simulink model "Discrete_time_PID"  (R2024b)
settings: Solver=ode45  StartTime=0.0  StopTime=10  RelTol=1e-3
values from neighbouring files (symbols this model uses):
  B_C = (gbox.N * mot.Ke)/drv.dcgain    [Init.m]
  Beq = 1.223604206496999e-06    (= 1.2236042065e-06)    [code_ali.m]
  den = [(TL+Ts) -TL]    [Init.m]
  F_C = mot.Req/(drv.dcgain * mot.Kt * gbox.N)    [Init.m]
  I_C = (gbox.N * mot.Req * Jeq_hat)/(drv.dcgain * mot.Kt)    [Init.m]
  Kw = 1/Tw*0.05    (= 1.66666666667)    [Init.m]
  num = [1 -1]    [Init.m]
  Ts = 50e-3    (= 0.05)    [Init.m]
undefined symbols (not defined in the file or in its folder): den_EX, den_FE, den_T, DiscIntNeverNeededParam, gbox, Kd, Ki, Kp, num_EX, num_FE, num_T, rpm2rads, sens, tau_sf
libraries: simulink x1
settings Model: Creator=Banaan  LastModifiedBy=lucag

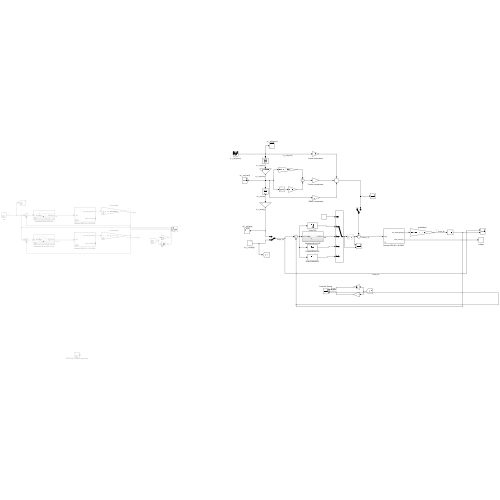
[thumbnail: Simulink's stored preview of the top-level diagram]
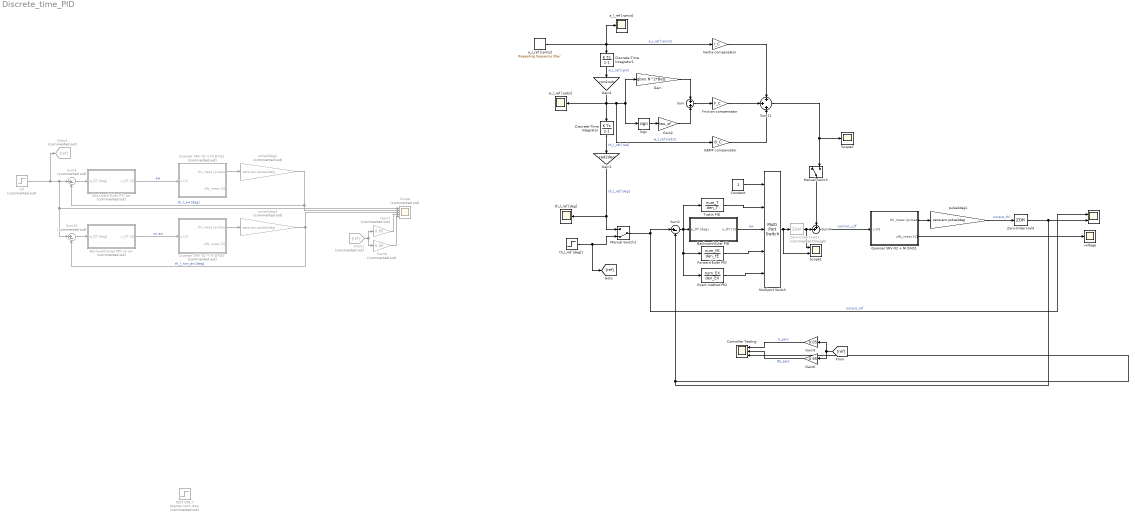
== system Discrete_time_PID ==
  " " : Scope  NumInputPorts=2
  " a_l_ref [rpm/s]" : Scope
  " th_l_ref [deg]" : Scope
  " w_l_ref [rad/s]" : Scope
  BEMF compensator : Gain  Gain=B_C
  Backward Euler PID : Subsystem
  Backward Euler PID aw : Subsystem  Commented=on
  Backward Euler PID no aw : Subsystem  Commented=on
  Constant : Constant
  Controller Testing : Scope  NumInputPorts=3
  Discrete-Time Integrator : DiscreteIntegrator  SampleTime=Ts  ICPrevOutput=DiscIntNeverNeededParam  ICPrevScaledInput=DiscIntNeverNeededParam
  Discrete-Time Integrator1 : DiscreteIntegrator  SampleTime=Ts  ICPrevOutput=DiscIntNeverNeededParam  ICPrevScaledInput=DiscIntNeverNeededParam
  Exact method PID : DiscreteTransferFcn  Numerator=num_EX  Denominator=den_EX
  Forward Euler PID : DiscreteTransferFcn  Numerator=num_FE  Denominator=den_FE
  Friction compensator : Gain  Gain=F_C
  From1 : From  Commented=on  GotoTag=ref
  Gain : Gain  Gain=gbox.N^2*Beq
  Gain1 : Gain  Gain=rad2deg
  Gain2 : Gain  Gain=tau_sf
  Gain3 : Gain  Gain=0.05
  Gain4 : Gain  Gain=rpm2rads
  Gain6 : Gain  Gain=0.95
  Gain7 : Gain  Commented=on  Gain=0.95
  Gain8 : Gain  Commented=on  Gain=0.05
  Goto1 : Goto  Commented=on  GotoTag=ref
  Inertia compensator : Gain  Gain=I_C
  Manual Switch : ManualSwitch
  Manual Switch1 : ManualSwitch  CurrentSetting=0
  Multiport Switch : MultiPortSwitch  DataPortOrder=Specify indices  DataPortIndices={1,2,3,4}  SaturateOnIntegerOverflow=off  InputSameDT=off
  Quanser SRV-02 + NI DAQ1 : Subsystem  mask(Quanser SRV-02 (with inertial load) + NI DAQ){Ts=0.001, fricType=Coulomb + viscous}
      mask prompts: Ts "NI DAQ Sample Time:"; fricType "Friction model"
      mask help: Quanser SRV-02 (with inertial load) + NI DAQ model.
      mask init:
      | %%  Sensors data
      | 
      | %   shunt resistor
      | sens.curr.Rs = 0.5;                         %   resistance [Ohm]   
      | sens.curr.uRs_std = 0.01;                   %   voltage noise standard dev [V]                           
      | sens.curr.uRs_var = sens.curr.uRs_std^2;	%   voltage noise variance [V^2]
      | 
      | %   Hewlett-Packard HEDS-5540#A06 optical encoder
      | sens.enc.ppr = 500*4;                       %   pulses per rotation
      | sens.enc.pulse2deg = 360/sens.enc.ppr;      %   [pulses] -> [deg]
      | sens.enc.pulse2rad = 2*pi/sens.enc.ppr;     %   [pulses] -> [rad]
      | sens.enc.deg2pulse = sens.enc.ppr/360;      %   [deg] -> [pulses]
      | sens.enc.rad2pulse = sens.enc.ppr/2/pi;     %   [rad] -> [pulses]
      | 
      | 
      | %%  Data acquisition board (daq) data
      | 
      | %   NI PCI-6221 DAC data
      | daq.dac.bits = 16;                                  %   resolution (bits)
      | daq.dac.fs   = 10;                                  %   full scale 
      | daq.dac.q    = 2*daq.dac.fs/(2^daq.dac.bits-1);     %	quantization
      | 
      | %   NI PCI-6221 ADC data
      | daq.adc.bits = 16;                                  %   resolution (bits)
      | daq.adc.fs   = 10;                                  %   full scale (as set in SLDRT Analog Input block)
      | daq.adc.q    = 2*daq.adc.fs/(2^daq.adc.bits-1);     %   quantization
      mask Help:
      | Riccardo Antonello (antonello@dei.unipd.it)
      | 
      | April 24, 2020
      | 
      | Dept. of Information Engineering, University of Padova
      mask TypeOptions fricType: Coulomb + viscous | Karnopp
  Quanser SRV-02 + NI DAQ2 : Subsystem  Commented=on  mask(Quanser SRV-02 (with inertial load) + NI DAQ){Ts=0.001, fricType=Coulomb + viscous}
      mask prompts: Ts "NI DAQ Sample Time:"; fricType "Friction model"
      mask help: Quanser SRV-02 (with inertial load) + NI DAQ model.
      mask init: same as Discrete_time_PID/Quanser SRV-02 + NI DAQ1
      mask Help:
      | Riccardo Antonello (antonello@dei.unipd.it)
      | 
      | April 24, 2020
      | 
      | Dept. of Information Engineering, University of Padova
      mask TypeOptions fricType: Coulomb + viscous | Karnopp
  Quanser SRV-02 + NI DAQ3 : Subsystem  Commented=on  mask(Quanser SRV-02 (with inertial load) + NI DAQ){Ts=0.001, fricType=Coulomb + viscous}
      mask prompts: Ts "NI DAQ Sample Time:"; fricType "Friction model"
      mask help: Quanser SRV-02 (with inertial load) + NI DAQ model.
      mask init: same as Discrete_time_PID/Quanser SRV-02 + NI DAQ1
      mask Help:
      | Riccardo Antonello (antonello@dei.unipd.it)
      | 
      | April 24, 2020
      | 
      | Dept. of Information Engineering, University of Padova
      mask TypeOptions fricType: Coulomb + viscous | Karnopp
  Scope : Scope  Commented=on  NumInputPorts=5
  Scope1 : Scope  NumInputPorts=2
  Scope2 : Scope
  Sign : Signum
  Sum : Sum  Inputs=+|+
  Sum10 : Sum  Commented=on  Inputs=|+-
  Sum11 : Sum  Inputs=+|+|+
  Sum2 : Sum  Inputs=|+-
  Sum4 : Sum  Inputs=++|
  Sum9 : Sum  Commented=on  Inputs=|+-
  TEST ONLY degree-input step : Step  Commented=on  After=360  SampleTime=0
  Tustin PID : DiscreteTransferFcn  Numerator=num_T  Denominator=den_T
  Zero-Order Hold : ZeroOrderHold  SampleTime=Ts
  Zero-Order Hold1 : ZeroOrderHold  Commented=through  SampleTime=Ts
  a_l_ref [rpm/s] : simulink/Sources/Repeating Sequence Stair  OutValues=[900 0 -900 -900 0 900]  tsamp=0.5  OutMin=[]  OutMax=[]  OutDataTypeStr=double  OutputDataTypeScalingMode=double  OutDataType=fixdt(0,8)  ConRadixGroup=Best Precision: Vector-wise  OutScaling=2^-12
  pulse2deg1 : Gain  Gain=sens.enc.pulse2deg
  pulse2deg2 : Gain  Commented=on  Gain=sens.enc.pulse2deg
  pulse2deg3 : Gain  Commented=on  Gain=sens.enc.pulse2deg
  ref : Step  Commented=on  After=500  SampleTime=0
  th_l_ref [deg]1 : Step  After=360  SampleTime=0
  voltage : Scope
  wires:
  Gain3/1 -> Controller Testing/1  "5_perc"
  Quanser SRV-02 + NI DAQ1/1(thl_meas [pulses]) -> pulse2deg1/1
  Gain6/1 -> Controller Testing/2  "95_perc"
  Quanser SRV-02 + NI DAQ1/2(uRs_meas [V]) -> voltage/1
  pulse2deg1/1 -> Zero-Order Hold/1  "output_thl"
  Sum4/1 -> Quanser SRV-02 + NI DAQ1/1(u [V])  "control_u_ff"
  Sum9/1 -> Backward Euler PID aw/1(e_DT [deg])
  Quanser SRV-02 + NI DAQ2/1(thl_meas [pulses]) -> pulse2deg2/1
  Quanser SRV-02 + NI DAQ3/1(thl_meas [pulses]) -> pulse2deg3/1
  Sum10/1 -> Backward Euler PID no aw/1(e_DT [deg])
  pulse2deg2/1 -> Scope/2, Sum9/2  "th_l_aw [deg]"
  pulse2deg3/1 -> Scope/3, Sum10/2  "th_l_non_aw [deg]"
  ref/1 -> Goto1/1, Sum10/1, Scope/1, Sum9/1
  Manual Switch/1 -> Sum4/1
  Manual Switch1/1 -> Sum2/1, " "/1  "output_ref"
  th_l_ref [deg]1/1 -> [ref], Manual Switch1/2
  [ref] -> Gain6/1, Gain3/1
  From1/1 -> Gain8/1, Gain7/1
  Gain7/1 -> Scope/4
  Gain8/1 -> Scope/5
  Friction compensator/1 -> Sum11/2
  Sum/1 -> Friction compensator/1
  a_l_ref [rpm/s]/1 -> Discrete-Time Integrator1/1, " a_l_ref [rpm/s]"/1, Inertia compensator/1  "a_l_ref [rpm/s]"
  Gain/1 -> Sum/1
  Inertia compensator/1 -> Sum11/1
  Sum11/1 -> Scope2/1, Manual Switch/2
  Discrete-Time Integrator1/1 -> Gain4/1  "w_l_ref [rpm]"
  Gain4/1 -> BEMF compensator/1, Sign/1, Gain/1, Discrete-Time Integrator/1, " w_l_ref [rad/s]"/1  "w_l_ref [rad/s]"
  Discrete-Time Integrator/1 -> Gain1/1  "th_l_ref [rad]"
  BEMF compensator/1 -> Sum11/3
  Gain2/1 -> Sum/2
  Sign/1 -> Gain2/1
  Gain1/1 -> Manual Switch1/1, " th_l_ref [deg]"/1  "th_l_ref [deg]"
  Forward Euler PID/1 -> Multiport Switch/4
  Constant/1 -> Multiport Switch/1
  Multiport Switch/1 -> Scope1/2, Zero-Order Hold1/1
  Sum2/1 -> Exact method PID/1, Forward Euler PID/1, Tustin PID/1, Backward Euler PID/1(e_DT [deg])
  Backward Euler PID/1(u_DT [V]) -> Multiport Switch/3  "aw"
  Backward Euler PID aw/1(u_DT [V]) -> Quanser SRV-02 + NI DAQ2/1(u [V])  "aw"
  Backward Euler PID no aw/1(u_DT [V]) -> Quanser SRV-02 + NI DAQ3/1(u [V])  "no aw"
  Zero-Order Hold/1 -> " "/2, Sum2/2, Controller Testing/3
  Exact method PID/1 -> Multiport Switch/5
  Zero-Order Hold1/1 -> Scope1/1, Sum4/2
  Tustin PID/1 -> Multiport Switch/2

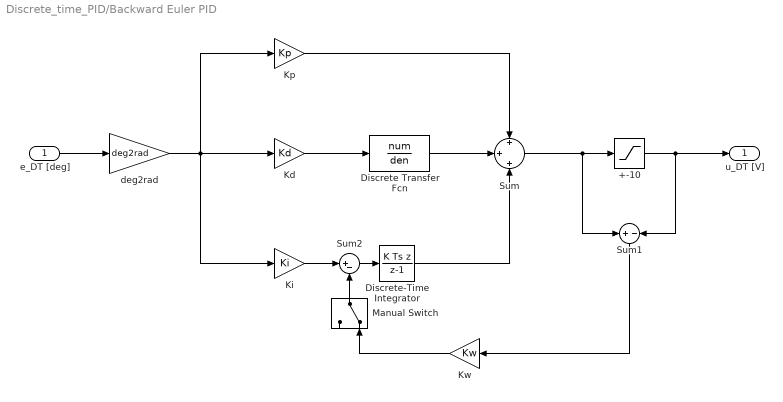
== system Discrete_time_PID/Backward Euler PID ==
  e_DT [deg] : Inport
  +-10 : Saturate  UpperLimit=10  LowerLimit=-10
  Discrete Transfer Fcn : DiscreteTransferFcn  Numerator=num  Denominator=den
  Discrete-Time Integrator : DiscreteIntegrator  IntegratorMethod=Integration: Backward Euler  gainval=Ts  SampleTime=Ts  ICPrevOutput=DiscIntNeverNeededParam  ICPrevScaledInput=DiscIntNeverNeededParam
  Kd : Gain  Gain=Kd
  Ki : Gain  Gain=Ki
  Kp : Gain  Gain=Kp
  Kw : Gain  Gain=Kw
  Manual Switch : ManualSwitch  CurrentSetting=0
  Sum : Sum  Inputs=+|+|+
  Sum1 : Sum  Inputs=+|-
  Sum2 : Sum  Inputs=|+-
  deg2rad : Gain  Gain=deg2rad
  u_DT [V] : Outport
  wires:
  e_DT [deg]/1 -> deg2rad/1
  deg2rad/1 -> Kp/1, Ki/1, Kd/1
  Ki/1 -> Sum2/1
  Kp/1 -> Sum/1
  Discrete-Time Integrator/1 -> Sum/3
  Kd/1 -> Discrete Transfer Fcn/1
  Discrete Transfer Fcn/1 -> Sum/2
  Sum/1 -> Sum1/1, +-10/1
  Sum1/1 -> Kw/1
  Kw/1 -> Manual Switch/2
  +-10/1 -> u_DT [V]/1, Sum1/2
  Manual Switch/1 -> Sum2/2
  Sum2/1 -> Discrete-Time Integrator/1

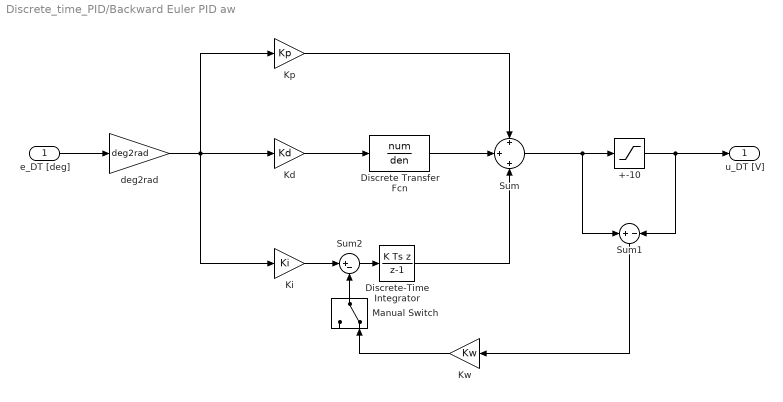
== system Discrete_time_PID/Backward Euler PID aw ==
  e_DT [deg] : Inport
  +-10 : Saturate  UpperLimit=10  LowerLimit=-10
  Discrete Transfer Fcn : DiscreteTransferFcn  Numerator=num  Denominator=den
  Discrete-Time Integrator : DiscreteIntegrator  IntegratorMethod=Integration: Backward Euler  gainval=Ts  SampleTime=Ts  ICPrevOutput=DiscIntNeverNeededParam  ICPrevScaledInput=DiscIntNeverNeededParam
  Kd : Gain  Gain=Kd
  Ki : Gain  Gain=Ki
  Kp : Gain  Gain=Kp
  Kw : Gain  Gain=Kw
  Manual Switch : ManualSwitch  CurrentSetting=0
  Sum : Sum  Inputs=+|+|+
  Sum1 : Sum  Inputs=+|-
  Sum2 : Sum  Inputs=|+-
  deg2rad : Gain  Gain=deg2rad
  u_DT [V] : Outport
  wires:
  Sum2/1 -> Discrete-Time Integrator/1
  Manual Switch/1 -> Sum2/2
  +-10/1 -> Sum1/2, u_DT [V]/1
  Kw/1 -> Manual Switch/2
  Sum1/1 -> Kw/1
  Sum/1 -> +-10/1, Sum1/1
  Discrete Transfer Fcn/1 -> Sum/2
  Kd/1 -> Discrete Transfer Fcn/1
  Discrete-Time Integrator/1 -> Sum/3
  Kp/1 -> Sum/1
  Ki/1 -> Sum2/1
  deg2rad/1 -> Kd/1, Ki/1, Kp/1
  e_DT [deg]/1 -> deg2rad/1

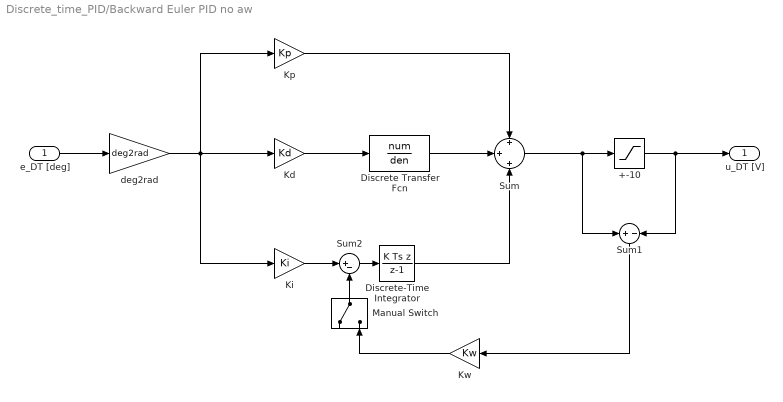
== system Discrete_time_PID/Backward Euler PID no aw ==
  e_DT [deg] : Inport
  +-10 : Saturate  UpperLimit=10  LowerLimit=-10
  Discrete Transfer Fcn : DiscreteTransferFcn  Numerator=num  Denominator=den
  Discrete-Time Integrator : DiscreteIntegrator  IntegratorMethod=Integration: Backward Euler  gainval=Ts  SampleTime=Ts  ICPrevOutput=DiscIntNeverNeededParam  ICPrevScaledInput=DiscIntNeverNeededParam
  Kd : Gain  Gain=Kd
  Ki : Gain  Gain=Ki
  Kp : Gain  Gain=Kp
  Kw : Gain  Gain=Kw
  Manual Switch : ManualSwitch
  Sum : Sum  Inputs=+|+|+
  Sum1 : Sum  Inputs=+|-
  Sum2 : Sum  Inputs=|+-
  deg2rad : Gain  Gain=deg2rad
  u_DT [V] : Outport
  wires:
  e_DT [deg]/1 -> deg2rad/1
  deg2rad/1 -> Kp/1, Ki/1, Kd/1
  Ki/1 -> Sum2/1
  Kp/1 -> Sum/1
  Discrete-Time Integrator/1 -> Sum/3
  Kd/1 -> Discrete Transfer Fcn/1
  Discrete Transfer Fcn/1 -> Sum/2
  Sum/1 -> Sum1/1, +-10/1
  Sum1/1 -> Kw/1
  Kw/1 -> Manual Switch/2
  +-10/1 -> u_DT [V]/1, Sum1/2
  Manual Switch/1 -> Sum2/2
  Sum2/1 -> Discrete-Time Integrator/1

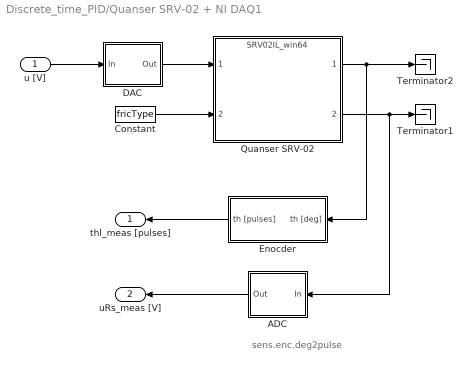
== system Discrete_time_PID/Quanser SRV-02 + NI DAQ1 ==
  note: sens.enc.deg2pulse
  u [V] : Inport
  ADC : Subsystem
  Constant : Constant  Value=fricType
  DAC : Subsystem
  Enocder : Subsystem
  Quanser SRV-02 : ModelReference  ModelNameDialog=SRV02IL_win64.slxp  ModelReferenceVersion=1.44  CopyOfModelProtected=on
  Terminator1 : Terminator
  Terminator2 : Terminator
  thl_meas [pulses] : Outport
  uRs_meas [V] : Outport  Port=2
  wires:
  Enocder/1(th [pulses]) -> thl_meas [pulses]/1
  ADC/1(Out) -> uRs_meas [V]/1
  DAC/1(Out) -> Quanser SRV-02/1
  Quanser SRV-02/2 -> ADC/1(In), Terminator1/1
  u [V]/1 -> DAC/1(In)
  Quanser SRV-02/1 -> Enocder/1(th [deg]), Terminator2/1
  Constant/1 -> Quanser SRV-02/2

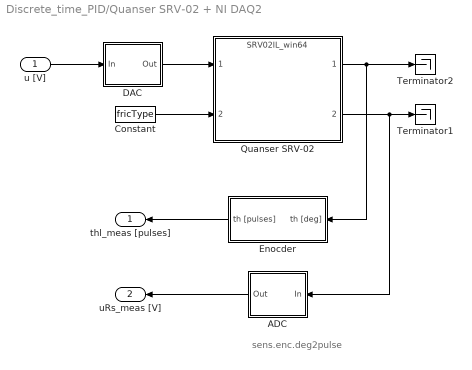
== system Discrete_time_PID/Quanser SRV-02 + NI DAQ2 ==
  note: sens.enc.deg2pulse
  u [V] : Inport
  ADC : Subsystem
  Constant : Constant  Value=fricType
  DAC : Subsystem
  Enocder : Subsystem
  Quanser SRV-02 : ModelReference  ModelNameDialog=SRV02IL_win64.slxp  ModelReferenceVersion=1.44  CopyOfModelProtected=on
  Terminator1 : Terminator
  Terminator2 : Terminator
  thl_meas [pulses] : Outport
  uRs_meas [V] : Outport  Port=2
  wires:
  Constant/1 -> Quanser SRV-02/2
  Quanser SRV-02/1 -> Terminator2/1, Enocder/1(th [deg])
  u [V]/1 -> DAC/1(In)
  Quanser SRV-02/2 -> Terminator1/1, ADC/1(In)
  DAC/1(Out) -> Quanser SRV-02/1
  ADC/1(Out) -> uRs_meas [V]/1
  Enocder/1(th [pulses]) -> thl_meas [pulses]/1

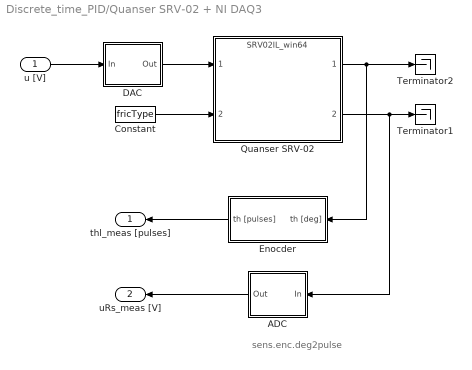
== system Discrete_time_PID/Quanser SRV-02 + NI DAQ3 ==
  note: sens.enc.deg2pulse
  u [V] : Inport
  ADC : Subsystem
  Constant : Constant  Value=fricType
  DAC : Subsystem
  Enocder : Subsystem
  Quanser SRV-02 : ModelReference  ModelNameDialog=SRV02IL_win64.slxp  ModelReferenceVersion=1.44  CopyOfModelProtected=on
  Terminator1 : Terminator
  Terminator2 : Terminator
  thl_meas [pulses] : Outport
  uRs_meas [V] : Outport  Port=2
  wires:
  Enocder/1(th [pulses]) -> thl_meas [pulses]/1
  ADC/1(Out) -> uRs_meas [V]/1
  DAC/1(Out) -> Quanser SRV-02/1
  Quanser SRV-02/2 -> ADC/1(In), Terminator1/1
  u [V]/1 -> DAC/1(In)
  Quanser SRV-02/1 -> Enocder/1(th [deg]), Terminator2/1
  Constant/1 -> Quanser SRV-02/2

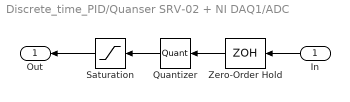
== system Discrete_time_PID/Quanser SRV-02 + NI DAQ1/ADC ==
  In : Inport
  Quantizer : Quantizer  QuantizationInterval=daq.adc.q
  Saturation : Saturate  UpperLimit=daq.adc.fs  LowerLimit=-daq.adc.fs
  Zero-Order Hold : ZeroOrderHold  SampleTime=Ts
  Out : Outport
  wires:
  Saturation/1 -> Out/1
  In/1 -> Zero-Order Hold/1
  Quantizer/1 -> Saturation/1
  Zero-Order Hold/1 -> Quantizer/1

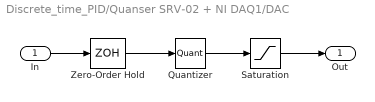
== system Discrete_time_PID/Quanser SRV-02 + NI DAQ1/DAC ==
  In : Inport
  Quantizer : Quantizer  QuantizationInterval=daq.dac.q
  Saturation : Saturate  UpperLimit=daq.dac.fs  LowerLimit=-daq.dac.fs
  Zero-Order Hold : ZeroOrderHold  SampleTime=Ts
  Out : Outport
  wires:
  Quantizer/1 -> Saturation/1
  In/1 -> Zero-Order Hold/1
  Zero-Order Hold/1 -> Quantizer/1
  Saturation/1 -> Out/1

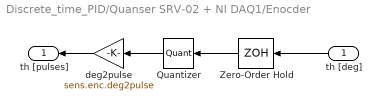
== system Discrete_time_PID/Quanser SRV-02 + NI DAQ1/Enocder ==
  th [deg] : Inport
  Quantizer : Quantizer  QuantizationInterval=sens.enc.pulse2deg
  Zero-Order Hold : ZeroOrderHold  SampleTime=Ts
  deg2pulse : Gain  Gain=sens.enc.deg2pulse
  th [pulses] : Outport
  wires:
  Quantizer/1 -> deg2pulse/1
  th [deg]/1 -> Zero-Order Hold/1
  Zero-Order Hold/1 -> Quantizer/1
  deg2pulse/1 -> th [pulses]/1

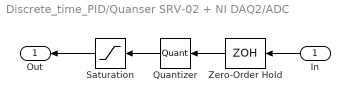
== system Discrete_time_PID/Quanser SRV-02 + NI DAQ2/ADC ==
  In : Inport
  Quantizer : Quantizer  QuantizationInterval=daq.adc.q
  Saturation : Saturate  UpperLimit=daq.adc.fs  LowerLimit=-daq.adc.fs
  Zero-Order Hold : ZeroOrderHold  SampleTime=Ts
  Out : Outport
  wires:
  Zero-Order Hold/1 -> Quantizer/1
  Quantizer/1 -> Saturation/1
  In/1 -> Zero-Order Hold/1
  Saturation/1 -> Out/1

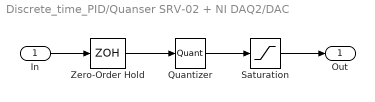
== system Discrete_time_PID/Quanser SRV-02 + NI DAQ2/DAC ==
  In : Inport
  Quantizer : Quantizer  QuantizationInterval=daq.dac.q
  Saturation : Saturate  UpperLimit=daq.dac.fs  LowerLimit=-daq.dac.fs
  Zero-Order Hold : ZeroOrderHold  SampleTime=Ts
  Out : Outport
  wires:
  Saturation/1 -> Out/1
  Zero-Order Hold/1 -> Quantizer/1
  In/1 -> Zero-Order Hold/1
  Quantizer/1 -> Saturation/1

== system Discrete_time_PID/Quanser SRV-02 + NI DAQ2/Enocder ==
  th [deg] : Inport
  Quantizer : Quantizer  QuantizationInterval=sens.enc.pulse2deg
  Zero-Order Hold : ZeroOrderHold  SampleTime=Ts
  deg2pulse : Gain  Gain=sens.enc.deg2pulse
  th [pulses] : Outport
  wires:
  deg2pulse/1 -> th [pulses]/1
  Zero-Order Hold/1 -> Quantizer/1
  th [deg]/1 -> Zero-Order Hold/1
  Quantizer/1 -> deg2pulse/1

== system Discrete_time_PID/Quanser SRV-02 + NI DAQ3/ADC ==
  In : Inport
  Quantizer : Quantizer  QuantizationInterval=daq.adc.q
  Saturation : Saturate  UpperLimit=daq.adc.fs  LowerLimit=-daq.adc.fs
  Zero-Order Hold : ZeroOrderHold  SampleTime=Ts
  Out : Outport
  wires:
  Saturation/1 -> Out/1
  In/1 -> Zero-Order Hold/1
  Quantizer/1 -> Saturation/1
  Zero-Order Hold/1 -> Quantizer/1

== system Discrete_time_PID/Quanser SRV-02 + NI DAQ3/DAC ==
  In : Inport
  Quantizer : Quantizer  QuantizationInterval=daq.dac.q
  Saturation : Saturate  UpperLimit=daq.dac.fs  LowerLimit=-daq.dac.fs
  Zero-Order Hold : ZeroOrderHold  SampleTime=Ts
  Out : Outport
  wires:
  Quantizer/1 -> Saturation/1
  In/1 -> Zero-Order Hold/1
  Zero-Order Hold/1 -> Quantizer/1
  Saturation/1 -> Out/1

== system Discrete_time_PID/Quanser SRV-02 + NI DAQ3/Enocder ==
  th [deg] : Inport
  Quantizer : Quantizer  QuantizationInterval=sens.enc.pulse2deg
  Zero-Order Hold : ZeroOrderHold  SampleTime=Ts
  deg2pulse : Gain  Gain=sens.enc.deg2pulse
  th [pulses] : Outport
  wires:
  Quantizer/1 -> deg2pulse/1
  th [deg]/1 -> Zero-Order Hold/1
  Zero-Order Hold/1 -> Quantizer/1
  deg2pulse/1 -> th [pulses]/1
